simulink model "faultHandling_combined"  (R2018a)
settings: Solver=VariableStepAuto  StartTime=0.0  StopTime=100  FixedStep=1e-2  MaxStep=1e-1  MinStep=1e-6  RelTol=1e-9
undefined symbols (not defined in the file): b, I, I_wheel, K, k_e, k_t, kd, ki, kp, L, magnitude, R
libraries: aausat3_lib x30, dspindex x3, sharedutil x1, library x1
(part 1 of 2)
settings Model: Creator=media  LastModifiedBy=Daniel
settings SolverCC: ZeroCrossAlgorithm=Adaptive  AlgebraicLoopSolver=LineSearch
settings DebuggingCC: MaxConsecutiveZCsMsg=none

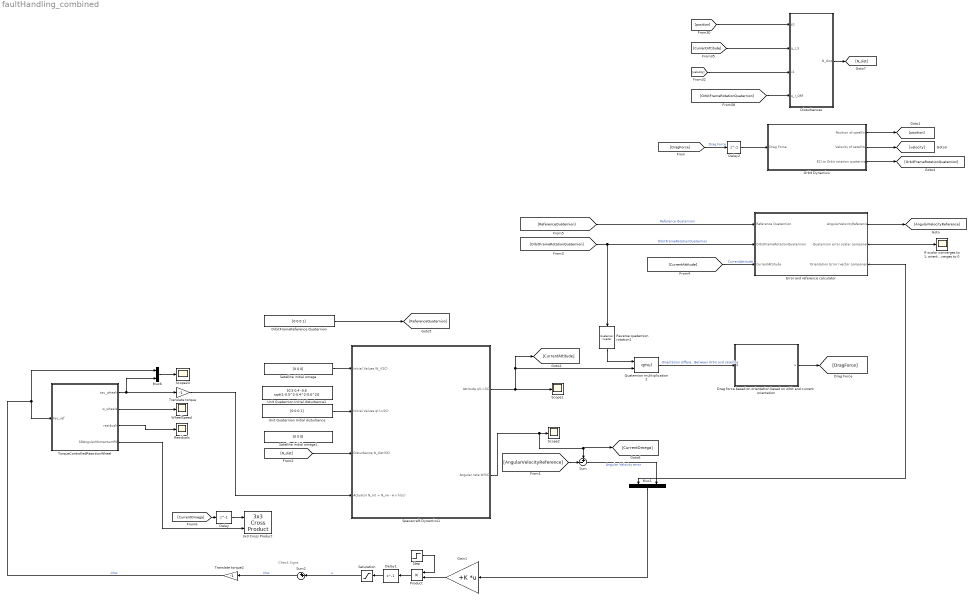
== system faultHandling_combined ==
  note: Check Signs
  3x3 Cross Product : sharedutil/3x3 Cross Product  aMode=aMode
      settings: SourceProductBaseCode=AE
  Delay : Delay  DelayLength=1  InitialCondition=[0;0;0]
  Delay1 : Delay  DelayLength=1  InitialCondition=[0;0;0]
  Delay2 : Delay  DelayLength=1  InitialCondition=0
  Disturbances : Subsystem
  Drag force based on orientation based on orbit and current orientation : Subsystem  TreatAsAtomicUnit=on
  Error and reference calculator : Subsystem
  Gain1 : Gain  Gain=+K  Multiplication=Matrix(K*u)
  "If scalar converges to 1, orientation error converges to 0" : Scope
  Mux1 : Mux  Inputs=2
  Mux6 : Mux  Inputs=2
  Orbit Dynamics : Subsystem
  OrbitFrameReference Quaternion : Constant  Value=[0 0 0 1]
  Product : Product
  Quaternion mulitiplication2 : S-Function  FunctionName=qmul  SFunctionDeploymentMode=off  EnableBusSupport=off
  Residuals : Scope
  Reverse quaternion rotation1 : aausat3_lib/Math Utilities/Quaternion operations/Vector rotation by q/Quaternion inverter
      settings: SourceProductName=AAUSAT3
  Satellite initial omega : Constant  Value=[0 0 0]
  Satellite initial omega1 : Constant  Value=[0 0 0]
  Saturation : Saturate  UpperLimit=2*10^-3  LowerLimit=-2*10^-3
  Scope1 : Scope
  Scope2 : Scope
  Scope24 : Scope
  Spacecraft Dynamics1 : Subsystem  AncestorBlock=spacecraft_dynamics2_lib/Spacecraft Dynamics
  Step : Step  Time=1000  Before=1  After=0  SampleTime=0
  Sum : Sum  Inputs=+-|
  Sum2 : Sum  Inputs=++|
  TorqueControlledReactionWheel : Subsystem
  Translate torque : Gain  Gain=-1
  Translate torque2 : Gain  Gain=-1
  Unit Quaternion Initial disturbance : Constant  Value=[0 0 0 1]
  Unit Quaternion Initial disturbance1 : Constant  Value=[0.5 0.4 -0.6 sqrt(1-0.5^2-0.4^2-0.6^2)]
  WheelSpeed : Scope
  wires:
  Satellite initial omega/1 -> Spacecraft Dynamics1/1(Initial Values W_i(SC))
  Unit Quaternion Initial disturbance/1 -> Spacecraft Dynamics1/2(Initial Values q(I->SC))
  Drag force based on orientation based on orbit and current orientation/1(u) -> [DragForce]
  Spacecraft Dynamics1/2(Angular rate W(SC)) -> [CurrentOmega], Sum/1, Scope2/1
  Quaternion mulitiplication2/1 -> Drag force based on orientation based on orbit and current orientation/1(q)  "Orientation difference Between Orbit and satellite"
  Spacecraft Dynamics1/1(Attitude q(I->SC)) -> [CurrentAttitude], Quaternion mulitiplication2/2, Scope1/1
  Reverse quaternion rotation1/1 -> Quaternion mulitiplication2/1
  [AngularVelocityReference] -> Sum/2
  Sum/1 -> Mux1/2  "Angular Velocity error"
  [velocity] -> Disturbances/3("v1 ")
  Disturbances/1(N_dist) -> [N_dist]
  [OrbitFrameRotationQuaternion] -> Disturbances/4(q_I_ORF)
  [position] -> Disturbances/1("p1 ")
  [CurrentAttitude] -> Disturbances/2("q_I_S ")
  [OrbitFrameRotationQuaternion] -> Reverse quaternion rotation1/1, Error and reference calculator/2(OrbitFrameRotationQuaternion)  "OrbitFrameRotationQuaternion"
  [DragForce] -> Delay2/1  "Drag Force"
  Orbit Dynamics/1(Position of satellite) -> [position]
  Orbit Dynamics/2(Velocity of satellite) -> [velocity]
  Orbit Dynamics/3(ECI to Orbit rotation quaternion) -> [OrbitFrameRotationQuaternion]
  [ReferenceQuaternion] -> Error and reference calculator/1(Reference Quaternion)  "Reference Quaternion"
  [CurrentAttitude] -> Error and reference calculator/3(CurrentAttitude)  "CurrentAttitude"
  Error and reference calculator/1(AngularVelocityReference) -> [AngularVelocityReference]
  Error and reference calculator/2(Quaternion error scalar component) -> "If scalar converges to 1, orientation error converges to 0"/1
  Error and reference calculator/3(Orientation Error (vector component)) -> Mux1/1
  TorqueControlledReactionWheel/2(w_wheels) -> WheelSpeed/1
  TorqueControlledReactionWheel/3(residuals) -> Residuals/1
  Mux6/1 -> Scope24/1
  OrbitFrameReference Quaternion/1 -> [ReferenceQuaternion]
  TorqueControlledReactionWheel/4(3DAngularMomentumRW) -> 3x3 Cross Product/2
  [CurrentOmega] -> Delay/1
  TorqueControlledReactionWheel/1(tau_wheels) -> Mux6/2, Translate torque/1
  Delay/1 -> 3x3 Cross Product/1
  Saturation/1 -> Sum2/2  "u"
  Translate torque2/1 -> Mux6/1, TorqueControlledReactionWheel/1("tau_ref ")  "-Nrw"
  Sum2/1 -> Translate torque2/1  "Nrw"
  Mux1/1 -> Gain1/1
  Gain1/1 -> Product/2
  Product/1 -> Delay1/1
  Step/1 -> Product/1
  [N_dist] -> Spacecraft Dynamics1/3(Disturbance N_dist(SC))
  Translate torque/1 -> Spacecraft Dynamics1/4(Actuator N_mt + N_rw - w x h(sc))
  Delay1/1 -> Saturation/1
  Delay2/1 -> Orbit Dynamics/1(Drag Force)

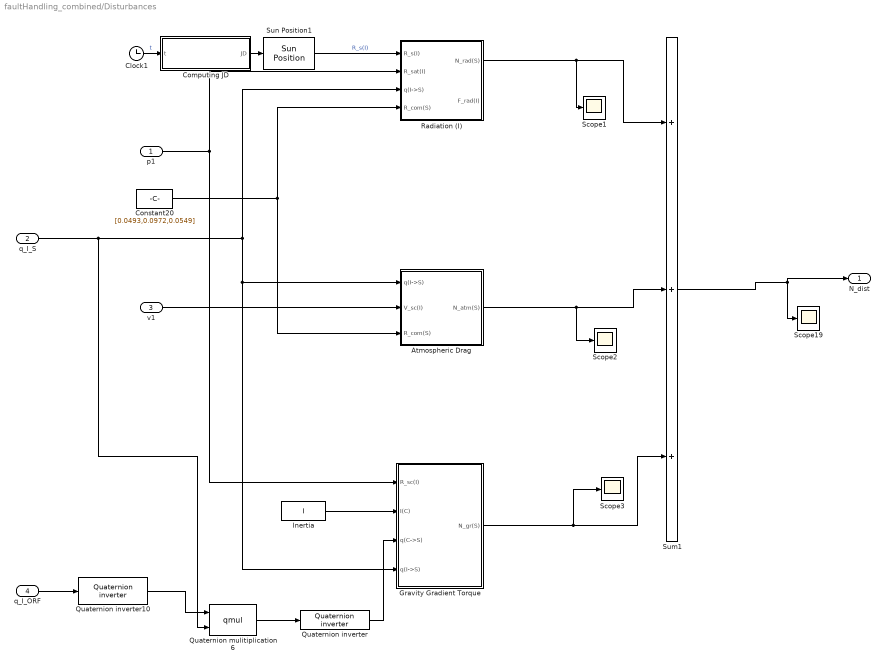
== system faultHandling_combined/Disturbances ==
  "p1 " : Inport
  "q_I_S " : Inport  Port=2
  "v1 " : Inport  Port=3
  q_I_ORF : Inport  Port=4
  Atmospheric Drag : Subsystem  AncestorBlock=aausat3_lib/Disturbances/Atmospheric  mask{Dim=[0.1,0.2,0.1], Cd=2, rho=5e-14}
      mask prompts: Dim "Satellite Dimension [x,y,z][m]:"; Cd "Drag Coefficient [-]:"; rho "Atmospheric Density [kg/m^3]:"
      mask help: Force and torque from the atmospheric drag acting on the satellite.
  Clock1 : Clock
      settings: Decimation=100
  Computing JD : MATLAB Function  TreatAsAtomicUnit=on
  Constant20 : Constant  Value=[0.0493,0.0972,0.0549]
  Gravity Gradient Torque : Subsystem  AncestorBlock=aausat3_lib/Disturbances/Gravity Gradient Torque  mask{G=6.672e-11, M_earth=5.9742e24}
      mask prompts: G "Gravitational Constant [m^3/kgs^2]:"; M_earth "Mass of the Earth [kg]:"
      mask help: Gravitational force applied by the Earth.
  Inertia : Constant  Value=I
  Quaternion inverter : aausat3_lib/Math Utilities/Quaternion operations/Quaternion inverter
      settings: SourceProductName=AAUSAT3
  Quaternion inverter10 : aausat3_lib/Math Utilities/Quaternion operations/Quaternion inverter
      settings: SourceProductName=AAUSAT3
  Quaternion mulitiplication6 : S-Function  FunctionName=qmul  SFunctionDeploymentMode=off  EnableBusSupport=off
  Radiation (I) : Subsystem  AncestorBlock=aausat3_lib/Disturbances/Radiation (I)  mask{Dim=[0.1,0.2,0.1], solar_m_flux=4.5565e-6, solar_absorb_coeff=1.5}
      mask prompts: Dim "Satellite Dimension [x,y,z][m]:"; solar_m_flux "Solar Momentum Flux [kg/ms^2]:"; solar_absorb_coeff "Absorbtion Coefficient [-]:"
      mask help: Solar force and torque acting on the satellite.
  Scope{1..3,19} (4 alike) : Scope
  Sum1 : Sum  Inputs=+++  SaturateOnIntegerOverflow=on
  Sun Position1 : aausat3_lib/Orbit and Ephemeris/Ephemeris/Sun Position
      settings: SourceProductName=AAUSAT3
  N_dist : Outport
  wires:
  Computing JD/1(JD) -> Sun Position1/1
  Sun Position1/1 -> Radiation (I)/1(R_s(I))  "R_s(I)"
  Clock1/1 -> Computing JD/1(t)  "t"
  Sum1/1 -> N_dist/1, Scope19/1
  "q_I_S "/1 -> Quaternion mulitiplication6/2, Radiation (I)/3(q(I->S)), Atmospheric Drag/1(q(I->S)), Gravity Gradient Torque/4(q(I->S))
  Atmospheric Drag/1(N_atm(S)) -> Scope2/1, Sum1/2
  Quaternion inverter10/1 -> Quaternion mulitiplication6/1
  q_I_ORF/1 -> Quaternion inverter10/1
  Quaternion mulitiplication6/1 -> Quaternion inverter/1
  Quaternion inverter/1 -> Gravity Gradient Torque/3(q(C->S))
  "v1 "/1 -> Atmospheric Drag/2(V_sc(I))
  Constant20/1 -> Radiation (I)/4(R_com(S)), Atmospheric Drag/3(R_com(S))
  Inertia/1 -> Gravity Gradient Torque/2(I(C))
  Radiation (I)/1(N_rad(S)) -> Scope1/1, Sum1/1
  Gravity Gradient Torque/1(N_gr(S)) -> Scope3/1, Sum1/3
  "p1 "/1 -> Gravity Gradient Torque/1(R_sc(I)), Radiation (I)/2(R_sat(I))

== system faultHandling_combined/Drag force based on orientation based on orbit and current orientation ==
  q : Inport
  Constant : Constant  Value=[1 0 0]
  Exposed area : aausat3_lib/Other Model Utilities/Exposed area  dim_sat_area=[0.1,0.1,0.1]
      settings: SourceProductName=AAUSAT3
  MATLAB Function : MATLAB Function  TreatAsAtomicUnit=on
  u : Outport
  wires:
  q/1 -> Exposed area/1
  Constant/1 -> Exposed area/2
  Exposed area/1 -> MATLAB Function/1(A)
  MATLAB Function/1(u) -> u/1

== system faultHandling_combined/Error and reference calculator ==
  Reference Quaternion : Inport
  OrbitFrameRotationQuaternion : Inport  Port=2
  CurrentAttitude : Inport  Port=3
  Avoiding Jumps In Quaternion : MATLAB Function  TreatAsAtomicUnit=on
  Demux2 : Demux
  Demux3 : Demux
  Derivative : Derivative
  Gain : Gain  Gain=2
  Mux : Mux  Inputs=3
  Mux2 : Mux  Inputs=3
  Quaternion mulitiplication{,1,3..5} (5 alike) : S-Function  FunctionName=qmul  SFunctionDeploymentMode=off  EnableBusSupport=off
  Reverse quaternion rotation : aausat3_lib/Math Utilities/Quaternion operations/Vector rotation by q/Quaternion inverter
      settings: SourceProductName=AAUSAT3
  Reverse quaternion rotation2 : aausat3_lib/Math Utilities/Quaternion operations/Vector rotation by q/Quaternion inverter
      settings: SourceProductName=AAUSAT3
  Reverse quaternion rotation4 : aausat3_lib/Math Utilities/Quaternion operations/Vector rotation by q/Quaternion inverter
      settings: SourceProductName=AAUSAT3
  AngularVelocityReference : Outport
  Quaternion error scalar component : Outport  Port=2
  Orientation Error (vector component) : Outport  Port=3
  wires:
  CurrentAttitude/1 -> Quaternion mulitiplication1/2
  OrbitFrameRotationQuaternion/1 -> Derivative/1, Reverse quaternion rotation2/1, Quaternion mulitiplication/1
  Quaternion mulitiplication1/1 -> Avoiding Jumps In Quaternion/1(q)  "Orientation Error Quaternion"
  Demux2/4 -> Quaternion error scalar component/1  "Quaternion error scalar component"
  Avoiding Jumps In Quaternion/1(q_continuous) -> Demux2/1
  Quaternion mulitiplication/1 -> Reverse quaternion rotation/1
  Reverse quaternion rotation/1 -> Quaternion mulitiplication1/1
  Demux2/2 -> Mux/2
  Demux2/3 -> Mux/3
  Derivative/1 -> Quaternion mulitiplication3/1
  Quaternion mulitiplication4/1 -> Quaternion mulitiplication5/1
  Reference Quaternion/1 -> Quaternion mulitiplication/2, Quaternion mulitiplication5/2, Reverse quaternion rotation4/1
  Gain/1 -> Quaternion mulitiplication4/2  "Pure Orbit Frame Quaternion"
  Quaternion mulitiplication3/1 -> Gain/1
  Demux3/1 -> Mux2/1
  Demux3/3 -> Mux2/3
  Demux3/2 -> Mux2/2
  Quaternion mulitiplication5/1 -> Demux3/1
  Reverse quaternion rotation4/1 -> Quaternion mulitiplication4/1
  Mux2/1 -> AngularVelocityReference/1  "AngularVelocityReference"
  Reverse quaternion rotation2/1 -> Quaternion mulitiplication3/2
  Demux2/1 -> Mux/1
  Mux/1 -> Orientation Error (vector component)/1  "Orientation Error (vector component)"

== system faultHandling_combined/Orbit Dynamics ==
  Drag Force : Inport
  Constant1 : Constant  Value=[0 0 0]
  Delay : Delay  DelayLength=1  InitialCondition=0
  Inertial frame to Orbit frame Rotation matrix : MATLAB Function  TreatAsAtomicUnit=on
  Initial velocity : Constant  Value=[0 7.5459e+03 0]
  Orbit frame distance : Constant  Value=[7*10^6 0 0]
  Satelllite 1 : S-Function  FunctionName=satDynamics_J2  Parameters=1, 5.9722*10^(24), 6.674*10^(-11), 6371009, 1.08262668*10^-3  SFunctionDeploymentMode=off  EnableBusSupport=off
  matrix_to_quaternion : MATLAB Function  TreatAsAtomicUnit=on
  Position of satellite : Outport
  Velocity of satellite : Outport  Port=2
  ECI to Orbit rotation quaternion : Outport  Port=3
  wires:
  Satelllite 1/2 -> Velocity of satellite/1, Inertial frame to Orbit frame Rotation matrix/2(v)  "Velocity of satellite"
  Drag Force/1 -> Satelllite 1/1
  Constant1/1 -> Satelllite 1/2  "Other Disturbances FORCES - but we only care about torques"
  Orbit frame distance/1 -> Satelllite 1/3  "Radius of orbit in meter"
  Initial velocity/1 -> Satelllite 1/4  "Initial velocity in orbit frame"
  Satelllite 1/1 -> Position of satellite/1, Inertial frame to Orbit frame Rotation matrix/1(p)  "Position of satellite"
  Inertial frame to Orbit frame Rotation matrix/1(rotation_matrix) -> matrix_to_quaternion/1(matrix)
  Delay/1 -> matrix_to_quaternion/2(q_prec)
  matrix_to_quaternion/1(q_I_ORF) -> ECI to Orbit rotation quaternion/1, Delay/1  "ECI to Orbit rotation quaternion"

== system faultHandling_combined/Spacecraft Dynamics1 ==
  Initial Values W_i(SC) : Inport
  Initial Values q(I->SC) : Inport  Port=2
  Disturbance N_dist(SC) : Inport  Port=3
  Actuator N_mt + N_rw - w x h(sc) : Inport  Port=4
  Dummy Nrw input : Constant  Value=[0 0 0]
  "Principal and Body frame is aligned, Principal frame  q(SC->P)" : Constant  Value=[0 0 0 1]
  Reaction wheel initial ang moment : Constant  Value=[0 0 0 ]
  Reverse quaternion rotation : aausat3_lib/Math Utilities/Quaternion operations/Vector rotation by q/Quaternion inverter
      settings: SourceProductName=AAUSAT3
  Rotation of q1 by q1 : aausat3_lib/Math Utilities/Quaternion operations/Rotation of q1 by q2
      settings: SourceProductName=AAUSAT3
  Rotation of q1 by q2 : aausat3_lib/Math Utilities/Quaternion operations/Rotation of q1 by q2
      settings: SourceProductName=AAUSAT3
  S-Function : S-Function  FunctionName=scdynamics3  SFunctionDeploymentMode=off  EnableBusSupport=off
  S-Function1 : S-Function  Commented=on  FunctionName=scdynamics2  SFunctionDeploymentMode=off  EnableBusSupport=off
  Spacecraft Inertia I(P) : Constant  Value=I
  Vector rotation by q{,2..4} (4 alike) : aausat3_lib/Math Utilities/Quaternion operations/Vector rotation by q
      settings: SourceProductName=AAUSAT3
  Attitude q(I->SC) : Outport
  Angular rate W(SC) : Outport  Port=2
  wires:
  S-Function/1 -> Vector rotation by q4/2
  S-Function/3 -> Rotation of q1 by q1/1
  Reaction wheel initial ang moment/1 -> S-Function/2
  Actuator N_mt + N_rw - w x h(sc)/1 -> Vector rotation by q2/2
  Vector rotation by q/1 -> S-Function/1
  Vector rotation by q2/1 -> S-Function/4
  Vector rotation by q3/1 -> S-Function/6
  Disturbance N_dist(SC)/1 -> Vector rotation by q3/2
  Dummy Nrw input/1 -> S-Function/5
  Rotation of q1 by q1/1 -> Attitude q(I->SC)/1
  Spacecraft Inertia I(P)/1 -> S-Function/7
  Rotation of q1 by q2/1 -> S-Function/3
  Vector rotation by q4/1 -> Angular rate W(SC)/1
  Initial Values q(I->SC)/1 -> Rotation of q1 by q2/1
  "Principal and Body frame is aligned, Principal frame  q(SC->P)"/1 -> Rotation of q1 by q2/2, Vector rotation by q/1, Vector rotation by q2/1, Vector rotation by q3/1, Reverse quaternion rotation/1
  Initial Values W_i(SC)/1 -> Vector rotation by q/2
  Reverse quaternion rotation/1 -> Vector rotation by q4/1, Rotation of q1 by q1/2

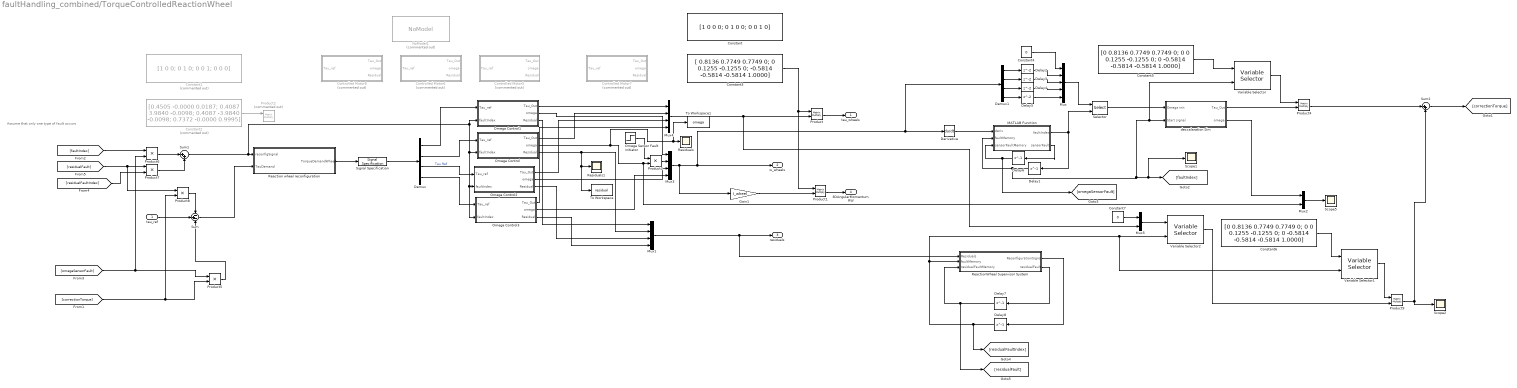
== system faultHandling_combined/TorqueControlledReactionWheel ==
  note: Assume that only one type of fault occurs
  "tau_ref " : Inport
  Constant : Constant  Value=[1 0 0 0; 0 1 0 0; 0 0 1 0]
  Constant1 : Constant  Commented=on  Value=[1 0 0; 0 1 0; 0 0 1; 0 0 0]
  Constant2 : Constant  Commented=on  Value=|
      | [0.4505   -0.0000    0.0187;
      |     0.4087    3.9840   -0.0098;
      |     0.4087   -3.9840   -0.0098;
      |     0.7372   -0.0000    0.9995]
  Constant3 : Constant  Value=|
      | [    0.8136    0.7749    0.7749         0;
      |          0    0.1255   -0.1255         0;
      |    -0.5814   -0.5814   -0.5814    1.0000]
  Constant4 : Constant  Value=0
  Constant5 : Constant  Value=|
      | [0    0.8136    0.7749    0.7749         0;
      |  0        0    0.1255   -0.1255         0;
      |  0  -0.5814   -0.5814   -0.5814    1.0000]
  Constant6 : Constant  Value=|
      | [0    0.8136    0.7749    0.7749         0;
      |  0        0    0.1255   -0.1255         0;
      |  0  -0.5814   -0.5814   -0.5814    1.0000]
  Constant7 : Constant  Value=0
  Controlled Motor5 : Subsystem  Commented=on
  Controlled Motor6 : Subsystem  Commented=on
  Controlled Motor7 : Subsystem  Commented=on
  Controlled Motor8 : Subsystem  Commented=on
  Delay{1,6..8} (4 alike) : Delay  DelayLength=1  InitialCondition=0
  Delay{2..5} (4 alike) : Delay  InitialCondition=0
  Demux : Demux
  Demux1 : Demux
  Derivative : Derivative
  Gain1 : Gain  Gain=I_wheel
  MATLAB Function : MATLAB Function  TreatAsAtomicUnit=on
  Mux : Mux  Inputs=5
  Mux1 : Mux
  Mux2 : Mux  Inputs=2
  Mux3 : Mux
  Mux4 : Mux
  Mux5 : Mux  Inputs=2
  NoModel1 : library/Reaction Wheel Models/NoModel  Commented=on
  Omega Control : Subsystem
  Omega Control1 : Subsystem
  Omega Control2 : Subsystem
  Omega Control3 : Subsystem
  Omega Sensor Fault initiator : Step  Time=1000  Before=1  After=0  SampleTime=0
  Product{,1,4,9} (4 alike) : Product  Multiplication=Matrix(*)
  Product2 : Product  Commented=on  Multiplication=Matrix(*)
  Product{3,5..8} (5 alike) : Product
  Reaction wheel reconfiguration : MATLAB Function  TreatAsAtomicUnit=on
  ReactionWheel Supervisor System : MATLAB Function  TreatAsAtomicUnit=on
  Residuals : Scope
  Residuals1 : Scope
  Scope1 : Scope
  Scope2 : Scope
  Scope5 : Scope
  Selector : Selector  IndexMode=Zero-based  InputPortWidth=5  IndexOptions=Index vector (port)  Indices=[1 3]  OutputSizes=1
  Signal Specification : SignalSpecification  Dimensions=4
  Sum : Sum  Inputs=-+-
  Sum1 : Sum  Inputs=|++
  Sum2 : Sum  Inputs=|++
  To Workspace : ToWorkspace  VariableName=residual  SaveFormat=Timeseries  SampleTime=-1
  To Workspace1 : ToWorkspace  VariableName=omega  SaveFormat=Timeseries  SampleTime=-1
  Variable Selector : dspindex/Variable Selector  NumInputs=1  rowsOrCols=Columns  IdxMode=Variable  Elements=[1 3]  ZerOneIdxMode=Zero-based  errmode=Clip Index  FillMode=on  FillValues=0
  Variable Selector1 : dspindex/Variable Selector  NumInputs=1  rowsOrCols=Columns  IdxMode=Variable  Elements=[1 3]  ZerOneIdxMode=Zero-based  errmode=Clip Index  FillMode=on  FillValues=0
  Variable Selector2 : dspindex/Variable Selector  NumInputs=1  rowsOrCols=Rows  IdxMode=Variable  Elements=[1 3]  ZerOneIdxMode=Zero-based  errmode=Clip Index  FillMode=on  FillValues=0
  deccalaration Sim : Subsystem
  tau_wheels : Outport
  w_wheels : Outport  Port=2
  residuals : Outport  Port=3
  3DAngularMomentumRW : Outport  Port=4
  wires:
  Demux/4 -> Omega Control3/1(Tau_ref)
  Omega Control3/1("Tau_Out ") -> Mux4/4
  Omega Control3/2(omega) -> Mux3/4
  Demux/3 -> Omega Control2/1(Tau_ref)  "Tau Ref"
  Demux/2 -> Omega Control/1(Tau_ref)
  Omega Control/1("Tau_Out ") -> Mux4/2
  Omega Control2/1("Tau_Out ") -> Mux4/3
  Omega Control1/2(omega) -> Mux3/1
  Omega Control2/2(omega) -> Mux3/3
  Omega Control1/3(Residual) -> Mux1/1
  Omega Control/3(Residual) -> To Workspace/1, Residuals1/1, Mux1/2
  Omega Control2/3(Residual) -> Mux1/3
  Omega Control3/3(Residual) -> Mux1/4
  Mux1/1 -> ReactionWheel Supervisor System/1(Residuals), residuals/1
  Omega Control1/1("Tau_Out ") -> Mux4/1
  Gain1/1 -> Product1/2
  Product/1 -> tau_wheels/1
  Product1/1 -> 3DAngularMomentumRW/1
  Demux/1 -> Omega Control1/1(Tau_ref)
  Constant3/1 -> Product1/1, Product/1
  Product3/1 -> Mux3/2
  Omega Control/2(omega) -> To Workspace1/1, Residuals/1, Mux2/2, Product3/2
  Derivative/1 -> MATLAB Function/1(deriv)
  Mux3/1 -> Gain1/1, Derivative/1, Demux1/1, w_wheels/1
  Selector/1 -> deccalaration Sim/1(Omega init)
  deccalaration Sim/2(omega) -> Mux2/1
  Demux1/1 -> Delay2/1
  Demux1/4 -> Delay5/1
  Demux1/3 -> Delay4/1
  Demux1/2 -> Delay3/1
  Delay5/1 -> Mux/5
  Delay4/1 -> Mux/4
  Delay3/1 -> Mux/3
  Delay2/1 -> Mux/2
  Constant4/1 -> Mux/1
  Mux/1 -> Selector/1
  Constant5/1 -> Variable Selector/1
  deccalaration Sim/1("Tau_Out ") -> Product4/2
  Constant2/1 -> Product2/1
  Sum1/1 -> Omega Control1/2(faultIndex), Omega Control2/2(faultIndex), Omega Control3/2(faultIndex), Omega Control/2(faultIndex), Reaction wheel reconfiguration/1(reconfigSignal)
  Variable Selector/1 -> Product4/1
  Signal Specification/1 -> Demux/1
  Reaction wheel reconfiguration/1(TorqueDemandWheel) -> Signal Specification/1
  Sum/1 -> Reaction wheel reconfiguration/2(TauDemand)
  Mux2/1 -> Scope5/1
  Omega Sensor Fault initiator/1 -> Product3/1
  MATLAB Function/2(sensorFault) -> Delay6/1
  Delay6/1 -> [omegaSensorFault], MATLAB Function/3(sensorFaultMemory)
  Delay1/1 -> MATLAB Function/2(faultMemory), Variable Selector/2, deccalaration Sim/2(Start signal), Scope1/1, [faultIndex]
  [correctionTorque] -> Product8/2, Product5/2
  [omegaSensorFault] -> Product5/1, Product6/2
  ReactionWheel Supervisor System/1(ReconfigurationSignal) -> Delay8/1
  MATLAB Function/1(faultIndex) -> Delay1/1, Selector/2
  Delay7/1 -> [residualFault], ReactionWheel Supervisor System/3(residualFaultMemory)
  ReactionWheel Supervisor System/2(residualFault) -> Delay7/1
  Delay8/1 -> [residualFaultIndex], ReactionWheel Supervisor System/2(faultMemory), Variable Selector1/2, Variable Selector2/2
  [faultIndex] -> Product6/1
  Product6/1 -> Sum1/1
  [residualFaultIndex] -> Product7/2
  [residualFault] -> Product8/1, Product7/1
  Product7/1 -> Sum1/2
  "tau_ref "/1 -> Sum/2
  Product5/1 -> Sum/3
  Product8/1 -> Sum/1
  Sum2/1 -> [correctionTorque]
  Product4/1 -> Sum2/1
  Constant6/1 -> Variable Selector1/1
  Variable Selector1/1 -> Product9/1
  Variable Selector2/1 -> Product9/2
  Mux4/1 -> Mux5/2, Product/2
  Product9/1 -> Sum2/2, Scope2/1
  Mux5/1 -> Variable Selector2/1
  Constant7/1 -> Mux5/1

== system faultHandling_combined/Disturbances/Atmospheric Drag ==
  q(I->S) : Inport
  V_sc(I) : Inport  Port=2
  R_com(S) : Inport  Port=3
  C_D : Constant  Value=Cd
  Cross Product : aausat3_lib/Math Utilities/Vector operations/Cross Product
      settings: SourceProductName=AAUSAT3
  Density : Constant  Value=rho
  Dimensions : Constant  Value=Dim
  Exposed area : aausat3_lib/Other Model Utilities/Exposed area  dim_sat_area=[0.1,0.2,0.1]
      settings: SourceProductName=AAUSAT3
  Gain : Gain  Gain=-1/2  SaturateOnIntegerOverflow=on  OutDataTypeStr=Inherit: Same as input  ParamDataTypeStr=Inherit: Same as input
  Gain1 : Gain  Gain=1/2  SaturateOnIntegerOverflow=on  OutDataTypeStr=Inherit: Same as input  ParamDataTypeStr=Inherit: Same as input
  Product{1..4} (4 alike) : Product  SaturateOnIntegerOverflow=on  OutDataTypeStr=Inherit: Same as first input
  Sum : Sum  Inputs=|-+
  To unit vector : aausat3_lib/Math Utilities/Vector operations/To unit vector
      settings: SourceProductName=AAUSAT3
  Vector rotation by q : aausat3_lib/Math Utilities/Quaternion operations/Vector rotation by q
      settings: SourceProductName=AAUSAT3
  math operation : Math  Operator=magnitude^2  SaturateOnIntegerOverflow=on
  N_atm(S) : Outport
  wires:
  Sum/1 -> Cross Product/1
  R_com(S)/1 -> Sum/1  "Center of Mass"
  Gain1/1 -> Sum/2  "Geometric Center"
  Dimensions/1 -> Gain1/1
  Vector rotation by q/1 -> Cross Product/2
  Gain/1 -> Vector rotation by q/2
  Product4/1 -> Gain/1
  q(I->S)/1 -> Exposed area/1, Vector rotation by q/1
  Density/1 -> Product3/2
  Product2/1 -> Product3/1
  Product1/1 -> Product2/2
  math operation/1 -> Product1/1
  To unit vector/1 -> Product1/2
  V_sc(I)/1 -> Exposed area/2, To unit vector/1, math operation/1
  Exposed area/1 -> Product2/1
  C_D/1 -> Product4/1
  Product3/1 -> Product4/2
  Cross Product/1 -> N_atm(S)/1

== system faultHandling_combined/Disturbances/Gravity Gradient Torque ==
  note: To principal frame
  R_sc(I) : Inport
  I(C) : Inport  Port=2
  q(C->S) : Inport  Port=3
  q(I->S) : Inport  Port=4
  " " : Subsystem
  3*GM : Gain  Gain=3*G*M_earth  SaturateOnIntegerOverflow=on  OutDataTypeStr=Inherit: Same as input  ParamDataTypeStr=Inherit: Same as input
  Constant : Constant  Value=3
  Constant1 : Constant  Value=[1 0 0;0 1 0;0 0 1]
  Constant2 : Constant  Value=[1 1 1]  VectorParams1D=off
  Cross Product : aausat3_lib/Math Utilities/Vector operations/Cross Product
      settings: SourceProductName=AAUSAT3
  Dot roduct : DotProduct  InputSameDT=on  OutDataTypeStr=Inherit: Inherit via internal rule
  Product : Product  Multiplication=Matrix(*)  SaturateOnIntegerOverflow=on  OutDataTypeStr=Inherit: Same as first input
  Product1 : Product  SaturateOnIntegerOverflow=on  OutDataTypeStr=Inherit: Same as first input
  Product2 : Product  Multiplication=Matrix(*)  SaturateOnIntegerOverflow=on  OutDataTypeStr=Inherit: Same as first input
  Product3 : Product  SaturateOnIntegerOverflow=on  OutDataTypeStr=Inherit: Same as first input
  R : Math  Operator=pow  SaturateOnIntegerOverflow=on
  To unit vector : aausat3_lib/Math Utilities/Vector operations/To unit vector
      settings: SourceProductName=AAUSAT3
  Vector rotation by q : aausat3_lib/Math Utilities/Quaternion operations/Vector rotation by q
      settings: SourceProductName=AAUSAT3
  inv : Math  Operator=reciprocal  SaturateOnIntegerOverflow=on
  inv1 : Math  Operator=sqrt  SaturateOnIntegerOverflow=on
  N_gr(S) : Outport
  wires:
  Cross Product/1 -> Vector rotation by q/2
  Dot roduct/1 -> inv1/1
  Product3/1 -> N_gr(S)/1
  R/1 -> 3*GM/1
  inv/1 -> R/1
  inv1/1 -> inv/1
  Constant/1 -> R/2
  To unit vector/1 -> Product/2, Cross Product/1
  q(C->S)/1 -> " "/1(q(C->SC)), Vector rotation by q/1
  q(I->S)/1 -> " "/2("q(I -> SC)")
  " "/1(R_sc(C)) -> To unit vector/1
  Product1/1 -> Product/1
  Product/1 -> Cross Product/2
  I(C)/1 -> Product2/1
  Constant2/1 -> Product2/2
  Product2/1 -> Product1/1
  Constant1/1 -> Product1/2
  R_sc(I)/1 -> Dot roduct/2, Dot roduct/1, " "/3(R_sc(I))
  3*GM/1 -> Product3/1
  Vector rotation by q/1 -> Product3/2

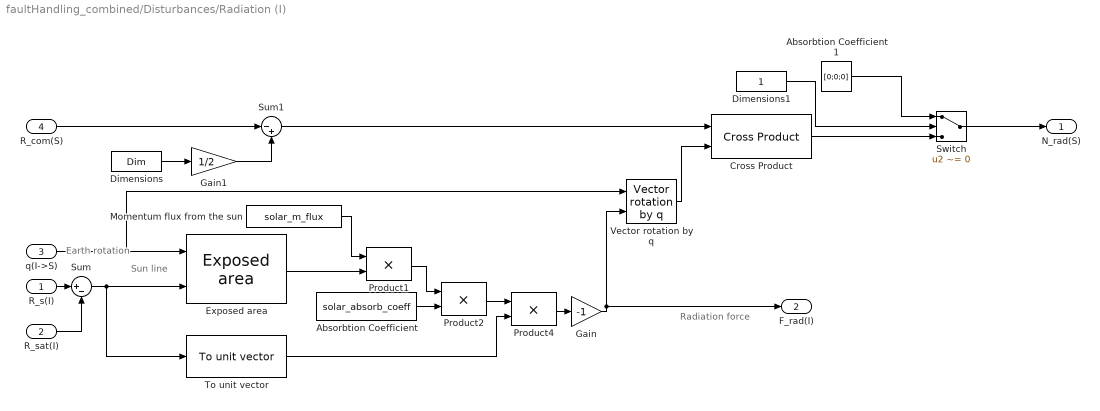
== system faultHandling_combined/Disturbances/Radiation (I) ==
  note: Sun line
  note: Earth rotation
  note: Radiation force
  R_s(I) : Inport
  R_sat(I) : Inport  Port=2
  q(I->S) : Inport  Port=3
  R_com(S) : Inport  Port=4
  Absorbtion Coefficient : Constant  Value=solar_absorb_coeff
  Absorbtion Coefficient1 : Constant  Value=[0;0;0]
  Cross Product : aausat3_lib/Math Utilities/Vector operations/Cross Product
      settings: SourceProductName=AAUSAT3
  Dimensions : Constant  Value=Dim
  Dimensions1 : Constant
  Exposed area : aausat3_lib/Other Model Utilities/Exposed area  dim_sat_area=[0.1,0.2,0.1]
      settings: SourceProductName=AAUSAT3
  Gain : Gain  Gain=-1  SaturateOnIntegerOverflow=on  OutDataTypeStr=Inherit: Same as input  ParamDataTypeStr=Inherit: Same as input
  Gain1 : Gain  Gain=1/2  SaturateOnIntegerOverflow=on  OutDataTypeStr=Inherit: Same as input  ParamDataTypeStr=Inherit: Same as input
  Momentum flux from the sun : Constant  Value=solar_m_flux
  Product1 : Product  SaturateOnIntegerOverflow=on  OutDataTypeStr=Inherit: Same as first input
  Product2 : Product  SaturateOnIntegerOverflow=on  OutDataTypeStr=Inherit: Same as first input
  Product4 : Product  SaturateOnIntegerOverflow=on  OutDataTypeStr=Inherit: Same as first input
  Sum : Sum  Inputs=|+-  SaturateOnIntegerOverflow=on
  Sum1 : Sum  Inputs=|-+
  Switch : Switch  Criteria=u2 ~= 0
  To unit vector : aausat3_lib/Math Utilities/Vector operations/To unit vector
      settings: SourceProductName=AAUSAT3
  Vector rotation by q : aausat3_lib/Math Utilities/Quaternion operations/Vector rotation by q
      settings: SourceProductName=AAUSAT3
  N_rad(S) : Outport
  F_rad(I) : Outport  Port=2
  wires:
  Absorbtion Coefficient1/1 -> Switch/1
  Switch/1 -> N_rad(S)/1
  R_s(I)/1 -> Sum/1
  R_sat(I)/1 -> Sum/2
  q(I->S)/1 -> Exposed area/1, Vector rotation by q/1
  Sum/1 -> Exposed area/2, To unit vector/1
  Product1/1 -> Product2/1
  Absorbtion Coefficient/1 -> Product2/2
  Product2/1 -> Product4/1
  To unit vector/1 -> Product4/2
  Product4/1 -> Gain/1
  Gain/1 -> Vector rotation by q/2, F_rad(I)/1
  Vector rotation by q/1 -> Cross Product/2
  Exposed area/1 -> Product1/2
  Momentum flux from the sun/1 -> Product1/1
  Cross Product/1 -> Switch/3
  Dimensions/1 -> Gain1/1
  R_com(S)/1 -> Sum1/1
  Gain1/1 -> Sum1/2
  Sum1/1 -> Cross Product/1
  Dimensions1/1 -> Switch/2

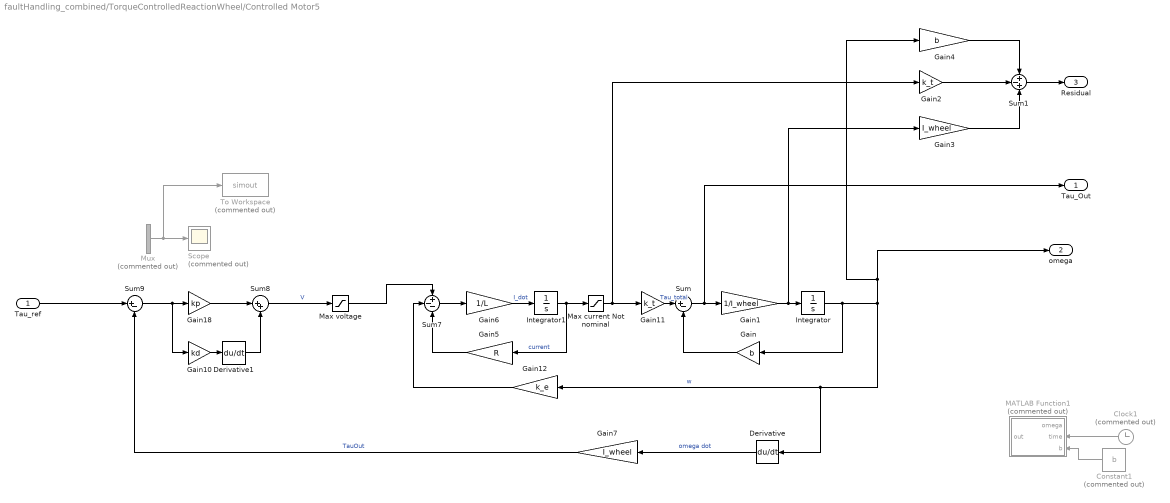
== system faultHandling_combined/TorqueControlledReactionWheel/Controlled Motor5 ==
  Tau_ref : Inport
  Clock1 : Clock  Commented=on
  Constant1 : Constant  Commented=on  Value=b
  Derivative : Derivative
  Derivative1 : Derivative
  Gain : Gain  Gain=b
  Gain1 : Gain  Gain=1/I_wheel
  Gain10 : Gain  Gain=kd
  Gain11 : Gain  Gain=k_t
  Gain12 : Gain  Gain=k_e
  Gain18 : Gain  Gain=kp
  Gain2 : Gain  Gain=k_t
  Gain3 : Gain  Gain=I_wheel
  Gain4 : Gain  Gain=b
  Gain5 : Gain  Gain=R
  Gain6 : Gain  Gain=1/L
  Gain7 : Gain  Gain=I_wheel
  Integrator : Integrator
  Integrator1 : Integrator
  MATLAB Function1 : MATLAB Function  Commented=on  TreatAsAtomicUnit=on
  Max current Not nominal : Saturate  UpperLimit=1.5  LowerLimit=-1.5
  Max voltage : Saturate  UpperLimit=6  LowerLimit=-6
  Mux : Mux  Commented=on  Inputs=2
  Scope : Scope  Commented=on
  Sum : Sum  Inputs=|+-
  Sum1 : Sum  Inputs=+-+
  Sum7 : Sum  Inputs=+--
  Sum8 : Sum  Inputs=|++
  Sum9 : Sum  Inputs=|+-
  To Workspace : ToWorkspace  Commented=on  VariableName=simout  SaveFormat=Timeseries  SampleTime=-1
  "Tau_Out " : Outport
  omega : Outport  Port=2
  Residual : Outport  Port=3
  wires:
  Max current Not nominal/1 -> Gain2/1, Gain11/1
  Derivative/1 -> Gain7/1  "omega dot"
  Gain18/1 -> Sum8/1
  Gain6/1 -> Integrator1/1  "I_dot"
  Sum7/1 -> Gain6/1
  Integrator/1 -> Gain/1, Gain4/1, omega/1, Derivative/1, Gain12/1  "w"
  Sum9/1 -> Gain10/1, Gain18/1
  Gain10/1 -> Derivative1/1
  Gain11/1 -> Sum/1  "Tau_total"
  Gain2/1 -> Sum1/2
  Gain4/1 -> Sum1/1
  Gain3/1 -> Sum1/3
  Sum1/1 -> Residual/1
  Sum8/1 -> Max voltage/1  "V"
  Tau_ref/1 -> Sum9/1
  Sum/1 -> "Tau_Out "/1, Gain1/1
  Gain1/1 -> Gain3/1, Integrator/1
  Max voltage/1 -> Sum7/1
  Gain12/1 -> Sum7/2
  Gain5/1 -> Sum7/3
  Integrator1/1 -> Gain5/1, Max current Not nominal/1  "current"
  Mux/1 -> To Workspace/1, Scope/1
  Constant1/1 -> MATLAB Function1/3(b)
  Clock1/1 -> MATLAB Function1/2(time)
  Gain/1 -> Sum/2
  Gain7/1 -> Sum9/2  "TauOut"
  Derivative1/1 -> Sum8/2

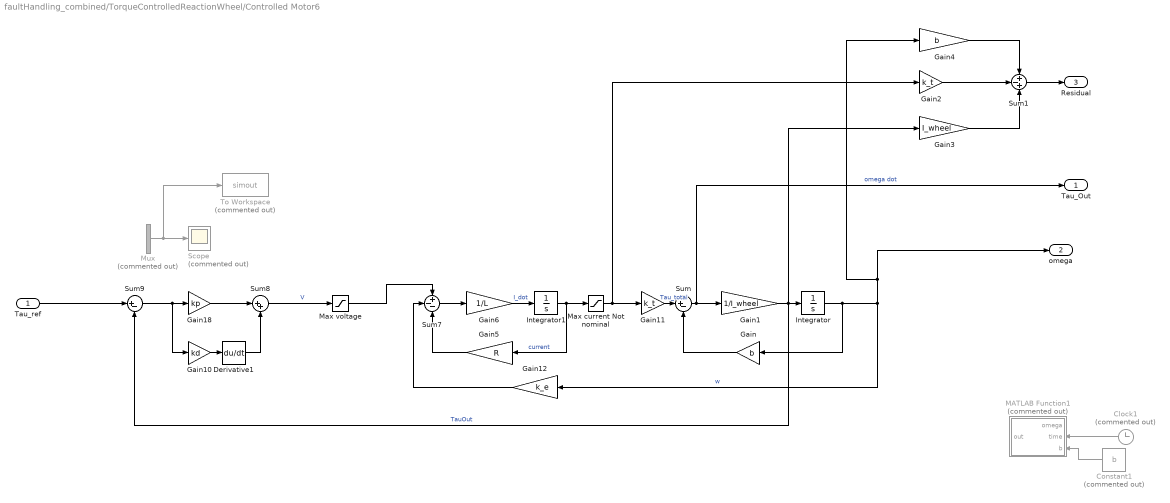
== system faultHandling_combined/TorqueControlledReactionWheel/Controlled Motor6 ==
  Tau_ref : Inport
  Clock1 : Clock  Commented=on
  Constant1 : Constant  Commented=on  Value=b
  Derivative1 : Derivative
  Gain : Gain  Gain=b
  Gain1 : Gain  Gain=1/I_wheel
  Gain10 : Gain  Gain=kd
  Gain11 : Gain  Gain=k_t
  Gain12 : Gain  Gain=k_e
  Gain18 : Gain  Gain=kp
  Gain2 : Gain  Gain=k_t
  Gain3 : Gain  Gain=I_wheel
  Gain4 : Gain  Gain=b
  Gain5 : Gain  Gain=R
  Gain6 : Gain  Gain=1/L
  Integrator : Integrator
  Integrator1 : Integrator
  MATLAB Function1 : MATLAB Function  Commented=on  TreatAsAtomicUnit=on
  Max current Not nominal : Saturate  UpperLimit=1.5  LowerLimit=-1.5
  Max voltage : Saturate  UpperLimit=6  LowerLimit=-6
  Mux : Mux  Commented=on  Inputs=2
  Scope : Scope  Commented=on
  Sum : Sum  Inputs=|+-
  Sum1 : Sum  Inputs=+-+
  Sum7 : Sum  Inputs=+--
  Sum8 : Sum  Inputs=|++
  Sum9 : Sum  Inputs=|+-
  To Workspace : ToWorkspace  Commented=on  VariableName=simout  SaveFormat=Timeseries  SampleTime=-1
  "Tau_Out " : Outport
  omega : Outport  Port=2
  Residual : Outport  Port=3
  wires:
  Max current Not nominal/1 -> Gain2/1, Gain11/1
  Sum/1 -> Gain1/1, "Tau_Out "/1  "omega dot"
  Gain18/1 -> Sum8/1
  Gain6/1 -> Integrator1/1  "I_dot"
  Sum7/1 -> Gain6/1
  Integrator/1 -> Gain/1, Gain4/1, omega/1, Gain12/1  "w"
  Sum9/1 -> Gain10/1, Gain18/1
  Gain10/1 -> Derivative1/1
  Gain11/1 -> Sum/1  "Tau_total"
  Gain2/1 -> Sum1/2
  Gain4/1 -> Sum1/1
  Gain3/1 -> Sum1/3
  Sum1/1 -> Residual/1
  Sum8/1 -> Max voltage/1  "V"
  Tau_ref/1 -> Sum9/1
  Max voltage/1 -> Sum7/1
  Gain12/1 -> Sum7/2
  Gain5/1 -> Sum7/3
  Integrator1/1 -> Gain5/1, Max current Not nominal/1  "current"
  Mux/1 -> To Workspace/1, Scope/1
  Constant1/1 -> MATLAB Function1/3(b)
  Clock1/1 -> MATLAB Function1/2(time)
  Gain/1 -> Sum/2
  Gain1/1 -> Sum9/2, Gain3/1, Integrator/1  "TauOut"
  Derivative1/1 -> Sum8/2

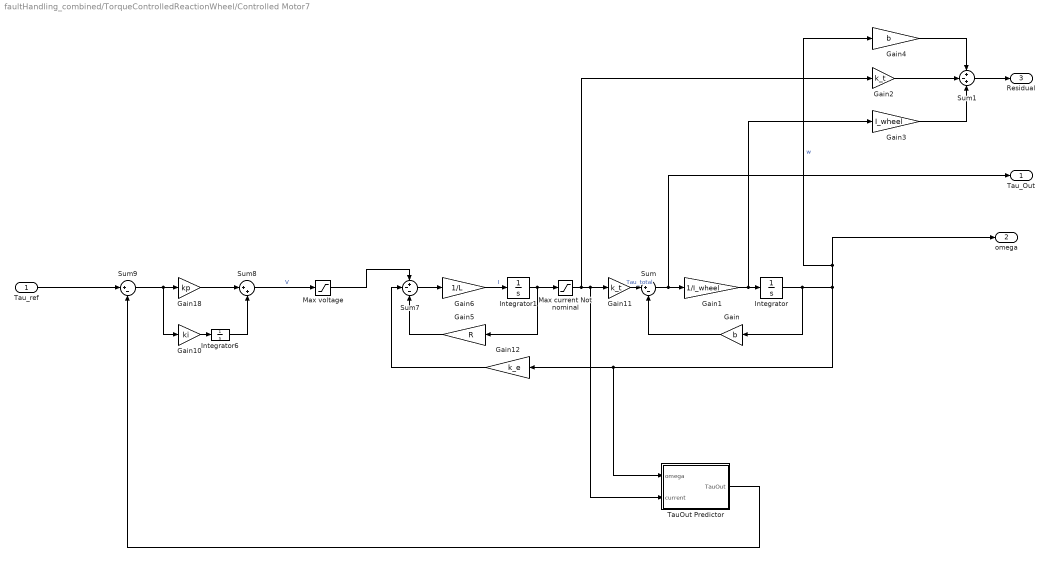
== system faultHandling_combined/TorqueControlledReactionWheel/Controlled Motor7 ==
  Tau_ref : Inport
  Gain : Gain  Gain=b
  Gain1 : Gain  Gain=1/I_wheel
  Gain10 : Gain  Gain=ki
  Gain11 : Gain  Gain=k_t
  Gain12 : Gain  Gain=k_e
  Gain18 : Gain  Gain=kp
  Gain2 : Gain  Gain=k_t
  Gain3 : Gain  Gain=I_wheel
  Gain4 : Gain  Gain=b
  Gain5 : Gain  Gain=R
  Gain6 : Gain  Gain=1/L
  Integrator : Integrator
  Integrator1 : Integrator
  Integrator6 : Integrator
  Max current Not nominal : Saturate  UpperLimit=1.5  LowerLimit=-1.5
  Max voltage : Saturate  UpperLimit=6  LowerLimit=-6
  Sum : Sum  Inputs=|+-
  Sum1 : Sum  Inputs=+-+
  Sum7 : Sum  Inputs=+--
  Sum8 : Sum  Inputs=|++
  Sum9 : Sum  Inputs=|+-
  TauOut Predictor : Subsystem
  "Tau_Out " : Outport
  omega : Outport  Port=2
  Residual : Outport  Port=3
  wires:
  Max current Not nominal/1 -> Gain2/1, Gain11/1, TauOut Predictor/2(current)
  TauOut Predictor/1(TauOut) -> Sum9/2
  Gain18/1 -> Sum8/1
  Integrator6/1 -> Sum8/2
  Gain6/1 -> Integrator1/1  "I"
  Sum7/1 -> Gain6/1
  Integrator/1 -> Gain/1, Gain4/1, omega/1, TauOut Predictor/1(omega), Gain12/1  "w"
  Sum9/1 -> Gain10/1, Gain18/1
  Gain10/1 -> Integrator6/1
  Gain11/1 -> Sum/1  "Tau_total"
  Gain2/1 -> Sum1/2
  Gain4/1 -> Sum1/1
  Gain3/1 -> Sum1/3
  Sum1/1 -> Residual/1
  Sum8/1 -> Max voltage/1  "V"
  Tau_ref/1 -> Sum9/1
  Gain/1 -> Sum/2
  Sum/1 -> "Tau_Out "/1, Gain1/1
  Gain1/1 -> Gain3/1, Integrator/1
  Max voltage/1 -> Sum7/1
  Gain12/1 -> Sum7/2
  Gain5/1 -> Sum7/3
  Integrator1/1 -> Gain5/1, Max current Not nominal/1

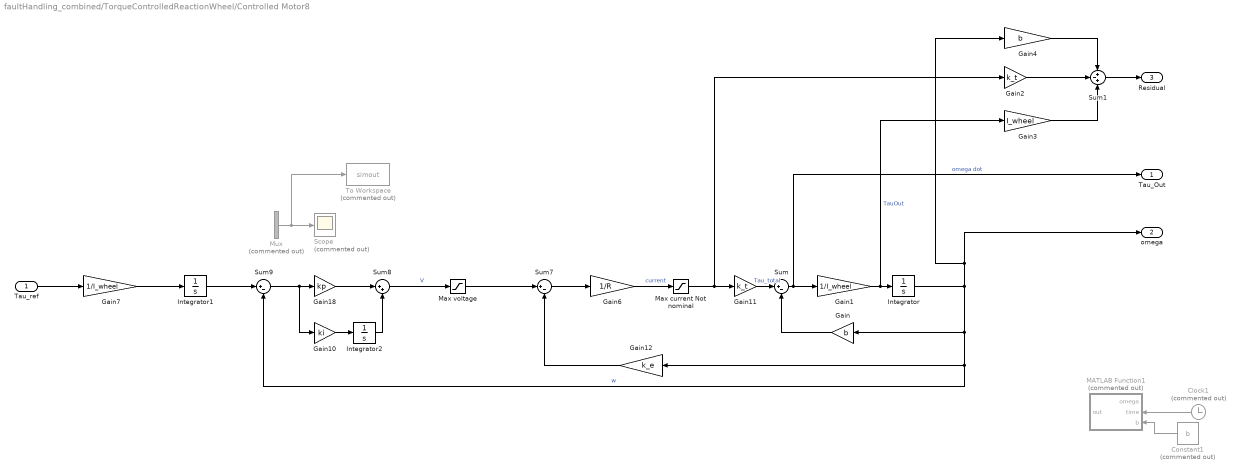
== system faultHandling_combined/TorqueControlledReactionWheel/Controlled Motor8 ==
  Tau_ref : Inport
  Clock1 : Clock  Commented=on
  Constant1 : Constant  Commented=on  Value=b
  Gain : Gain  Gain=b
  Gain1 : Gain  Gain=1/I_wheel
  Gain10 : Gain  Gain=ki
  Gain11 : Gain  Gain=k_t
  Gain12 : Gain  Gain=k_e
  Gain18 : Gain  Gain=kp
  Gain2 : Gain  Gain=k_t
  Gain3 : Gain  Gain=I_wheel
  Gain4 : Gain  Gain=b
  Gain6 : Gain  Gain=1/R
  Gain7 : Gain  Gain=1/I_wheel
  Integrator : Integrator
  Integrator1 : Integrator
  Integrator2 : Integrator
  MATLAB Function1 : MATLAB Function  Commented=on  TreatAsAtomicUnit=on
  Max current Not nominal : Saturate  UpperLimit=1.5  LowerLimit=-1.5
  Max voltage : Saturate  UpperLimit=6  LowerLimit=-6
  Mux : Mux  Commented=on  Inputs=2
  Scope : Scope  Commented=on
  Sum : Sum  Inputs=|+-
  Sum1 : Sum  Inputs=+-+
  Sum7 : Sum  Inputs=|+-
  Sum8 : Sum  Inputs=|++
  Sum9 : Sum  Inputs=|+-
  To Workspace : ToWorkspace  Commented=on  VariableName=simout  SaveFormat=Timeseries  SampleTime=-1
  "Tau_Out " : Outport
  omega : Outport  Port=2
  Residual : Outport  Port=3
  wires:
  Max current Not nominal/1 -> Gain2/1, Gain11/1
  Sum/1 -> Gain1/1, "Tau_Out "/1  "omega dot"
  Gain18/1 -> Sum8/1
  Integrator/1 -> Gain/1, Gain12/1, Sum9/2, Gain4/1, omega/1  "w"
  Sum9/1 -> Gain10/1, Gain18/1
  Gain10/1 -> Integrator2/1
  Gain11/1 -> Sum/1  "Tau_total"
  Gain2/1 -> Sum1/2
  Gain4/1 -> Sum1/1
  Gain3/1 -> Sum1/3
  Sum1/1 -> Residual/1
  Sum8/1 -> Max voltage/1  "V"
  Max voltage/1 -> Sum7/1
  Gain12/1 -> Sum7/2
  Gain6/1 -> Max current Not nominal/1  "current"
  Mux/1 -> To Workspace/1, Scope/1
  Constant1/1 -> MATLAB Function1/3(b)
  Clock1/1 -> MATLAB Function1/2(time)
  Gain/1 -> Sum/2
  Gain1/1 -> Gain3/1, Integrator/1  "TauOut"
  Integrator2/1 -> Sum8/2
  Tau_ref/1 -> Gain7/1
  Sum7/1 -> Gain6/1
  Gain7/1 -> Integrator1/1
  Integrator1/1 -> Sum9/1

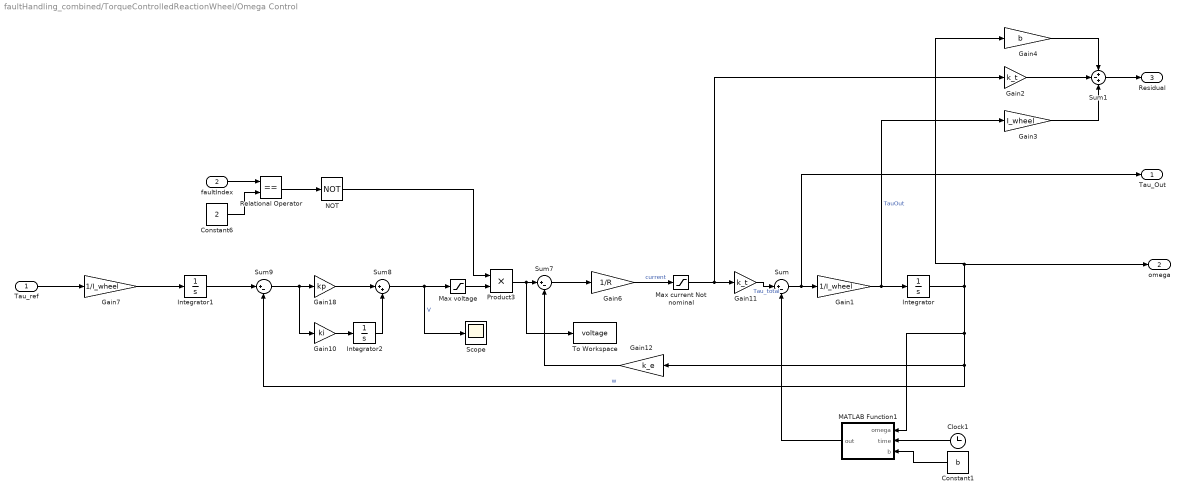
== system faultHandling_combined/TorqueControlledReactionWheel/Omega Control ==
  Tau_ref : Inport
  faultIndex : Inport  Port=2
  Clock1 : Clock
  Constant1 : Constant  Value=b
  Constant6 : Constant  Value=2
  Gain1 : Gain  Gain=1/I_wheel
  Gain10 : Gain  Gain=ki
  Gain11 : Gain  Gain=k_t
  Gain12 : Gain  Gain=k_e
  Gain18 : Gain  Gain=kp
  Gain2 : Gain  Gain=k_t
  Gain3 : Gain  Gain=I_wheel
  Gain4 : Gain  Gain=b
  Gain6 : Gain  Gain=1/R
  Gain7 : Gain  Gain=1/I_wheel
  Integrator : Integrator
  Integrator1 : Integrator
  Integrator2 : Integrator
  MATLAB Function1 : MATLAB Function  TreatAsAtomicUnit=on
  Max current Not nominal : Saturate  UpperLimit=1.5  LowerLimit=-1.5
  Max voltage : Saturate  UpperLimit=6  LowerLimit=-6
  NOT : Logic  Operator=NOT  IconShape=distinctive  AllPortsSameDT=off  OutDataTypeStr=boolean
  Product3 : Product
  Relational Operator : RelationalOperator  Operator===  OutDataTypeStr=boolean  ZeroCross=off  RndMeth=Simplest
  Scope : Scope
  Sum : Sum  Inputs=|+-
  Sum1 : Sum  Inputs=+-+
  Sum7 : Sum  Inputs=|+-
  Sum8 : Sum  Inputs=|++
  Sum9 : Sum  Inputs=|+-
  To Workspace : ToWorkspace  VariableName=voltage  SaveFormat=Timeseries  SampleTime=-1
  "Tau_Out " : Outport
  omega : Outport  Port=2
  Residual : Outport  Port=3
  wires:
  Max current Not nominal/1 -> Gain11/1, Gain2/1
  Sum/1 -> Gain1/1, "Tau_Out "/1
  Gain18/1 -> Sum8/1
  Integrator/1 -> MATLAB Function1/1(omega), Gain12/1, Sum9/2, Gain4/1, omega/1  "w"
  Sum9/1 -> Gain10/1, Gain18/1
  Gain10/1 -> Integrator2/1
  Gain11/1 -> Sum/1  "Tau_total"
  Gain2/1 -> Sum1/2
  Gain4/1 -> Sum1/1
  Gain3/1 -> Sum1/3
  Sum1/1 -> Residual/1
  Sum8/1 -> Scope/1, Max voltage/1  "V"
  Gain12/1 -> Sum7/2
  Gain6/1 -> Max current Not nominal/1  "current"
  Constant1/1 -> MATLAB Function1/3(b)
  Clock1/1 -> MATLAB Function1/2(time)
  MATLAB Function1/1(out) -> Sum/2
  Gain1/1 -> Gain3/1, Integrator/1  "TauOut"
  Integrator2/1 -> Sum8/2
  Tau_ref/1 -> Gain7/1
  Sum7/1 -> Gain6/1
  Gain7/1 -> Integrator1/1
  Integrator1/1 -> Sum9/1
  Product3/1 -> To Workspace/1, Sum7/1
  Max voltage/1 -> Product3/2
  NOT/1 -> Product3/1
  Relational Operator/1 -> NOT/1
  Constant6/1 -> Relational Operator/2
  faultIndex/1 -> Relational Operator/1

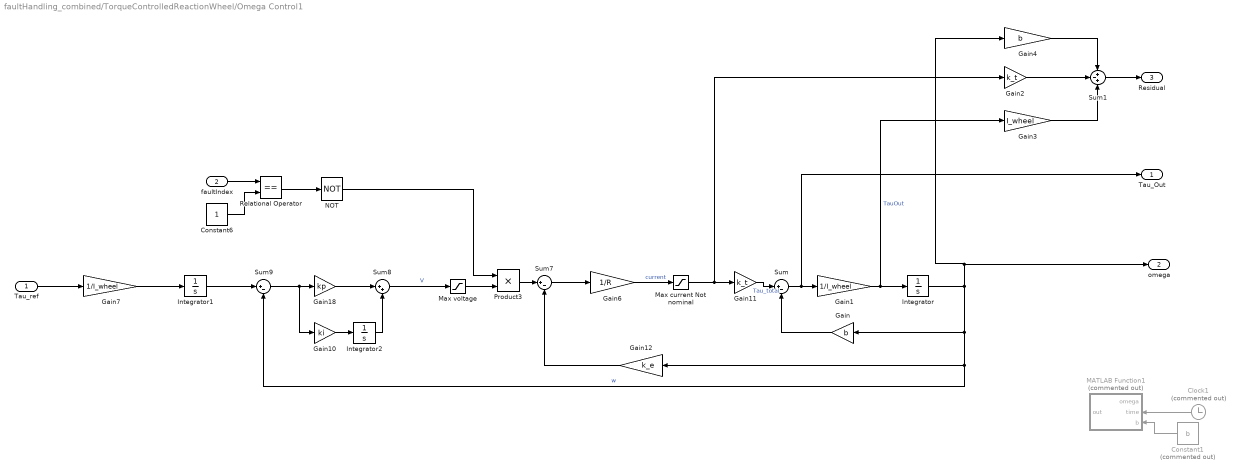
== system faultHandling_combined/TorqueControlledReactionWheel/Omega Control1 ==
  Tau_ref : Inport
  faultIndex : Inport  Port=2
  Clock1 : Clock  Commented=on
  Constant1 : Constant  Commented=on  Value=b
  Constant6 : Constant
  Gain : Gain  Gain=b
  Gain1 : Gain  Gain=1/I_wheel
  Gain10 : Gain  Gain=ki
  Gain11 : Gain  Gain=k_t
  Gain12 : Gain  Gain=k_e
  Gain18 : Gain  Gain=kp
  Gain2 : Gain  Gain=k_t
  Gain3 : Gain  Gain=I_wheel
  Gain4 : Gain  Gain=b
  Gain6 : Gain  Gain=1/R
  Gain7 : Gain  Gain=1/I_wheel
  Integrator : Integrator
  Integrator1 : Integrator
  Integrator2 : Integrator
  MATLAB Function1 : MATLAB Function  Commented=on  TreatAsAtomicUnit=on
  Max current Not nominal : Saturate  UpperLimit=1.5  LowerLimit=-1.5
  Max voltage : Saturate  UpperLimit=6  LowerLimit=-6
  NOT : Logic  Operator=NOT  IconShape=distinctive  AllPortsSameDT=off  OutDataTypeStr=boolean
  Product3 : Product
  Relational Operator : RelationalOperator  Operator===  OutDataTypeStr=boolean  ZeroCross=off  RndMeth=Simplest
  Sum : Sum  Inputs=|+-
  Sum1 : Sum  Inputs=+-+
  Sum7 : Sum  Inputs=|+-
  Sum8 : Sum  Inputs=|++
  Sum9 : Sum  Inputs=|+-
  "Tau_Out " : Outport
  omega : Outport  Port=2
  Residual : Outport  Port=3
  wires:
  Max current Not nominal/1 -> Gain11/1, Gain2/1
  Sum/1 -> Gain1/1, "Tau_Out "/1
  Gain18/1 -> Sum8/1
  Integrator/1 -> Gain/1, Gain12/1, Sum9/2, Gain4/1, omega/1  "w"
  Sum9/1 -> Gain10/1, Gain18/1
  Gain10/1 -> Integrator2/1
  Gain11/1 -> Sum/1  "Tau_total"
  Gain2/1 -> Sum1/2
  Gain4/1 -> Sum1/1
  Gain3/1 -> Sum1/3
  Sum1/1 -> Residual/1
  Sum8/1 -> Max voltage/1  "V"
  Gain12/1 -> Sum7/2
  Gain6/1 -> Max current Not nominal/1  "current"
  Constant1/1 -> MATLAB Function1/3(b)
  Clock1/1 -> MATLAB Function1/2(time)
  Gain/1 -> Sum/2
  Gain1/1 -> Gain3/1, Integrator/1  "TauOut"
  Integrator2/1 -> Sum8/2
  Tau_ref/1 -> Gain7/1
  Sum7/1 -> Gain6/1
  Gain7/1 -> Integrator1/1
  Integrator1/1 -> Sum9/1
  Product3/1 -> Sum7/1
  Max voltage/1 -> Product3/2
  NOT/1 -> Product3/1
  Relational Operator/1 -> NOT/1
  Constant6/1 -> Relational Operator/2
  faultIndex/1 -> Relational Operator/1

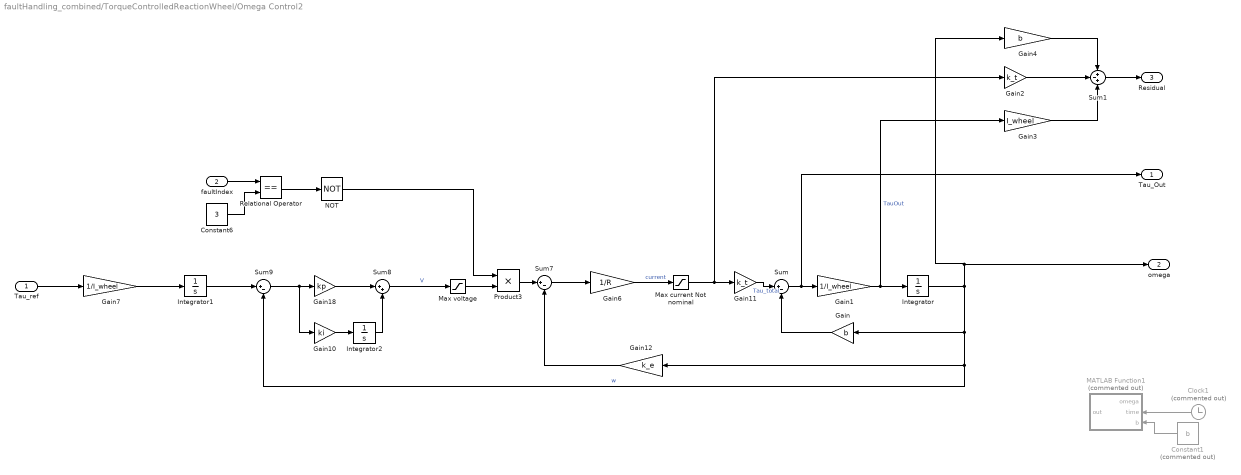
== system faultHandling_combined/TorqueControlledReactionWheel/Omega Control2 ==
  Tau_ref : Inport
  faultIndex : Inport  Port=2
  Clock1 : Clock  Commented=on
  Constant1 : Constant  Commented=on  Value=b
  Constant6 : Constant  Value=3
  Gain : Gain  Gain=b
  Gain1 : Gain  Gain=1/I_wheel
  Gain10 : Gain  Gain=ki
  Gain11 : Gain  Gain=k_t
  Gain12 : Gain  Gain=k_e
  Gain18 : Gain  Gain=kp
  Gain2 : Gain  Gain=k_t
  Gain3 : Gain  Gain=I_wheel
  Gain4 : Gain  Gain=b
  Gain6 : Gain  Gain=1/R
  Gain7 : Gain  Gain=1/I_wheel
  Integrator : Integrator
  Integrator1 : Integrator
  Integrator2 : Integrator
  MATLAB Function1 : MATLAB Function  Commented=on  TreatAsAtomicUnit=on
  Max current Not nominal : Saturate  UpperLimit=1.5  LowerLimit=-1.5
  Max voltage : Saturate  UpperLimit=6  LowerLimit=-6
  NOT : Logic  Operator=NOT  IconShape=distinctive  AllPortsSameDT=off  OutDataTypeStr=boolean
  Product3 : Product
  Relational Operator : RelationalOperator  Operator===  OutDataTypeStr=boolean  ZeroCross=off  RndMeth=Simplest
  Sum : Sum  Inputs=|+-
  Sum1 : Sum  Inputs=+-+
  Sum7 : Sum  Inputs=|+-
  Sum8 : Sum  Inputs=|++
  Sum9 : Sum  Inputs=|+-
  "Tau_Out " : Outport
  omega : Outport  Port=2
  Residual : Outport  Port=3
  wires:
  Max current Not nominal/1 -> Gain11/1, Gain2/1
  Sum/1 -> Gain1/1, "Tau_Out "/1
  Gain18/1 -> Sum8/1
  Integrator/1 -> Gain/1, Gain12/1, Sum9/2, Gain4/1, omega/1  "w"
  Sum9/1 -> Gain10/1, Gain18/1
  Gain10/1 -> Integrator2/1
  Gain11/1 -> Sum/1  "Tau_total"
  Gain2/1 -> Sum1/2
  Gain4/1 -> Sum1/1
  Gain3/1 -> Sum1/3
  Sum1/1 -> Residual/1
  Sum8/1 -> Max voltage/1  "V"
  Gain12/1 -> Sum7/2
  Gain6/1 -> Max current Not nominal/1  "current"
  Constant1/1 -> MATLAB Function1/3(b)
  Clock1/1 -> MATLAB Function1/2(time)
  Gain/1 -> Sum/2
  Gain1/1 -> Gain3/1, Integrator/1  "TauOut"
  Integrator2/1 -> Sum8/2
  Tau_ref/1 -> Gain7/1
  Sum7/1 -> Gain6/1
  Gain7/1 -> Integrator1/1
  Integrator1/1 -> Sum9/1
  Product3/1 -> Sum7/1
  Max voltage/1 -> Product3/2
  NOT/1 -> Product3/1
  Relational Operator/1 -> NOT/1
  Constant6/1 -> Relational Operator/2
  faultIndex/1 -> Relational Operator/1

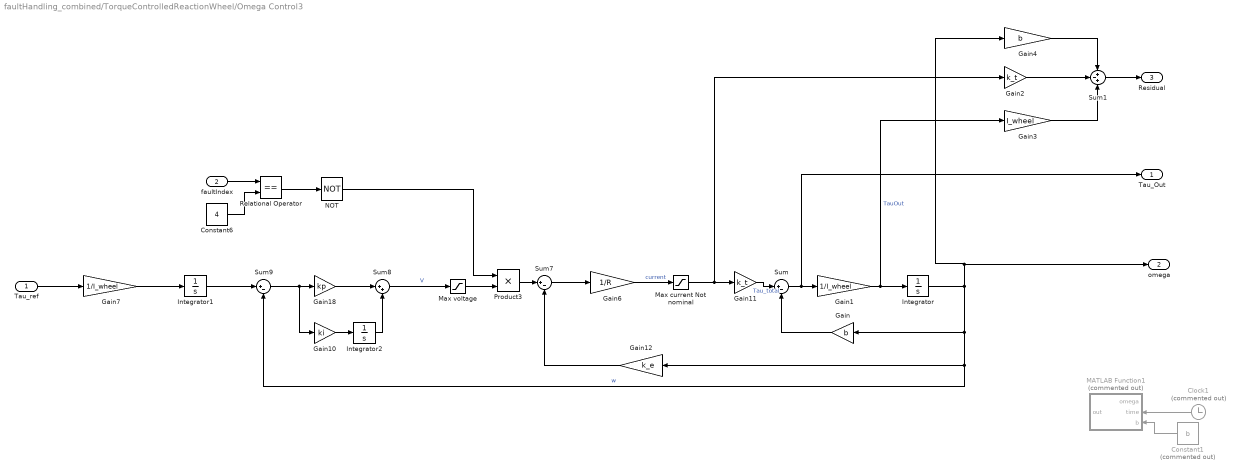
== system faultHandling_combined/TorqueControlledReactionWheel/Omega Control3 ==
  Tau_ref : Inport
  faultIndex : Inport  Port=2
  Clock1 : Clock  Commented=on
  Constant1 : Constant  Commented=on  Value=b
  Constant6 : Constant  Value=4
  Gain : Gain  Gain=b
  Gain1 : Gain  Gain=1/I_wheel
  Gain10 : Gain  Gain=ki
  Gain11 : Gain  Gain=k_t
  Gain12 : Gain  Gain=k_e
  Gain18 : Gain  Gain=kp
  Gain2 : Gain  Gain=k_t
  Gain3 : Gain  Gain=I_wheel
  Gain4 : Gain  Gain=b
  Gain6 : Gain  Gain=1/R
  Gain7 : Gain  Gain=1/I_wheel
  Integrator : Integrator
  Integrator1 : Integrator
  Integrator2 : Integrator
  MATLAB Function1 : MATLAB Function  Commented=on  TreatAsAtomicUnit=on
  Max current Not nominal : Saturate  UpperLimit=1.5  LowerLimit=-1.5
  Max voltage : Saturate  UpperLimit=6  LowerLimit=-6
  NOT : Logic  Operator=NOT  IconShape=distinctive  AllPortsSameDT=off  OutDataTypeStr=boolean
  Product3 : Product
  Relational Operator : RelationalOperator  Operator===  OutDataTypeStr=boolean  ZeroCross=off  RndMeth=Simplest
  Sum : Sum  Inputs=|+-
  Sum1 : Sum  Inputs=+-+
  Sum7 : Sum  Inputs=|+-
  Sum8 : Sum  Inputs=|++
  Sum9 : Sum  Inputs=|+-
  "Tau_Out " : Outport
  omega : Outport  Port=2
  Residual : Outport  Port=3
  wires:
  Max current Not nominal/1 -> Gain11/1, Gain2/1
  Sum/1 -> Gain1/1, "Tau_Out "/1
  Gain18/1 -> Sum8/1
  Integrator/1 -> Gain/1, Gain12/1, Sum9/2, Gain4/1, omega/1  "w"
  Sum9/1 -> Gain10/1, Gain18/1
  Gain10/1 -> Integrator2/1
  Gain11/1 -> Sum/1  "Tau_total"
  Gain2/1 -> Sum1/2
  Gain4/1 -> Sum1/1
  Gain3/1 -> Sum1/3
  Sum1/1 -> Residual/1
  Sum8/1 -> Max voltage/1  "V"
  Gain12/1 -> Sum7/2
  Gain6/1 -> Max current Not nominal/1  "current"
  Constant1/1 -> MATLAB Function1/3(b)
  Clock1/1 -> MATLAB Function1/2(time)
  Gain/1 -> Sum/2
  Gain1/1 -> Gain3/1, Integrator/1  "TauOut"
  Integrator2/1 -> Sum8/2
  Tau_ref/1 -> Gain7/1
  Sum7/1 -> Gain6/1
  Gain7/1 -> Integrator1/1
  Integrator1/1 -> Sum9/1
  Product3/1 -> Sum7/1
  Max voltage/1 -> Product3/2
  NOT/1 -> Product3/1
  Relational Operator/1 -> NOT/1
  Constant6/1 -> Relational Operator/2
  faultIndex/1 -> Relational Operator/1

== system faultHandling_combined/TorqueControlledReactionWheel/deccalaration Sim ==
  Omega init : Inport
  Start signal : Inport  Port=2
  Gain : Gain  Gain=b
  Gain1 : Gain  Gain=1/I_wheel
  Gain11 : Gain  Gain=k_t
  Gain12 : Gain  Gain=k_e
  Gain2 : Gain  Gain=-1
  Gain6 : Gain  Gain=1/R
  Integrator : Integrator  ExternalReset=rising  InitialConditionSource=external
  Max current Not nominal : Saturate  UpperLimit=1.5  LowerLimit=-1.5
  Sum : Sum  Inputs=|+-
  "Tau_Out " : Outport
  omega : Outport  Port=2
  wires:
  Max current Not nominal/1 -> Gain11/1
  Sum/1 -> Gain1/1, "Tau_Out "/1  "omega dot"
  Integrator/1 -> omega/1, Gain/1, Gain12/1  "w"
  Gain11/1 -> Sum/1  "Tau_total"
  Gain6/1 -> Max current Not nominal/1  "current"
  Gain/1 -> Sum/2
  Gain1/1 -> Integrator/1  "TauOut"
  Gain12/1 -> Gain2/1
  Omega init/1 -> Integrator/3
  Start signal/1 -> Integrator/2
  Gain2/1 -> Gain6/1

== system faultHandling_combined/Disturbances/Gravity Gradient Torque/  ==
  q(C->SC) : Inport
  "q(I -> SC)" : Inport  Port=2
  R_sc(I) : Inport  Port=3
  Quaternion inverter : aausat3_lib/Math Utilities/Quaternion operations/Quaternion inverter
      settings: SourceProductName=AAUSAT3
  Rotation of q1 by q2 : aausat3_lib/Math Utilities/Quaternion operations/Rotation of q1 by q2
      settings: SourceProductName=AAUSAT3
  To unit vector : aausat3_lib/Math Utilities/Vector operations/To unit vector
      settings: SourceProductName=AAUSAT3
  Vector rotation by q : aausat3_lib/Math Utilities/Quaternion operations/Vector rotation by q
      settings: SourceProductName=AAUSAT3
  R_sc(C) : Outport
  wires:
  "q(I -> SC)"/1 -> Rotation of q1 by q2/1
  q(C->SC)/1 -> Quaternion inverter/1
  Quaternion inverter/1 -> Rotation of q1 by q2/2
  R_sc(I)/1 -> To unit vector/1
  Rotation of q1 by q2/1 -> Vector rotation by q/1
  To unit vector/1 -> Vector rotation by q/2
  Vector rotation by q/1 -> R_sc(C)/1

== system faultHandling_combined/TorqueControlledReactionWheel/Controlled Motor7/TauOut Predictor ==
  omega : Inport
  current : Inport  Port=2
  Constant : Constant  Value=k_t
  Constant1 : Constant  Value=b
  Output torque estimator : MATLAB Function  TreatAsAtomicUnit=on
  TauOut : Outport
  wires:
  Output torque estimator/1(TauOut) -> TauOut/1
  Constant1/1 -> Output torque estimator/3(b)
  Constant/1 -> Output torque estimator/2(k_t)
  current/1 -> Output torque estimator/1(i)
  omega/1 -> Output torque estimator/4(omega)

== matlab function faultHandling_combined/Orbit Dynamics/matrix_to_quaternion ==
  data: matrix input; q_I_ORF output; q_prec input
function q_I_ORF = fcn(matrix,q_prec)

    tr = matrix(1,1) + matrix(2,2) + matrix(3,3);

    if( tr > 0 ) 
    	S = sqrt(tr+1.0) * 2;
        a = 0.25 * S;
        b = (matrix(3,2) - matrix(2,3)) / S;
        c = (matrix(1,3) - matrix(3,1)) / S; 
        d = (matrix(2,1) - matrix(1,2)) / S; 
    elseif( (matrix(1,1) > matrix(2,2) ) && ( matrix(1,1) > matrix(3,3) ) )
        S = sqrt(1.0 + matrix(1,1) - matrix(2,2) - matrix(3,3)) * 2;
        a = (matrix(3,2) - matrix(2,3)) / S;
        if( a < 0 )
            a = -a;
            S = -S;
        end
        b = 0.25 * S;
        c = (matrix(1,2) + matrix(2,1)) / S; 
        d = (matrix(1,3) + matrix(3,1)) / S; 
    elseif( matrix(2,2) > matrix(3,3) ) 
        S = sqrt(1.0 + matrix(2,2) - matrix(1,1) - matrix(3,3)) * 2;
        a = (matrix(1,3) - matrix(3,1)) / S;
        if( a < 0 )
            a = -a;
            S = -S;
        end
        b = (matrix(1,2) + matrix(2,1)) / S; 
        c = 0.25 * S;
        d = (matrix(2,3) + matrix(3,2)) / S; 
    else
        S = sqrt(1.0 + matrix(3,3) - matrix(1,1) - matrix(2,2)) * 2;
        a = (matrix(2,1) - matrix(1,2)) / S;
        if( a < 0 )
            a = -a;
            S = -S;
        end
        b = (matrix(1,3) + matrix(3,1)) / S;
        c = (matrix(2,3) + matrix(3,2)) / S;
        d = 0.25 * S;
    end
    
    q_I_ORF = [b,c,d,a]';
    
    
    if( (abs(q_I_ORF(1) - q_prec(1)) > 1) || (abs(q_I_ORF(2) - q_prec(2)) > 1) || (abs(q_I_ORF(3) - q_prec(3)) > 1) || (abs(q_I_ORF(4) - q_prec(4)) > 1) )
        q_I_ORF = - q_I_ORF;
    end
end

== matlab function faultHandling_combined/Orbit Dynamics/Inertial frame to Orbit frame Rotation matrix ==
  data: p input; rotation_matrix output; v input
function rotation_matrix = fcn(p,v)

    y_ORF = -p/norm(p);
    z_ORF = cross(v,y_ORF)/norm(cross(v,y_ORF));
    x_ORF = cross(y_ORF,z_ORF);
    
    rotation_matrix = [x_ORF, y_ORF, z_ORF];

== matlab function faultHandling_combined/Error and reference calculator/Avoiding Jumps In Quaternion ==
  data: q input; q_continuous output
function q_continuous = fcn(q)

   q_continuous = q;
   if(q(4) < 0)
       q_continuous = -q;
   end
   
    
end

== matlab function faultHandling_combined/TorqueControlledReactionWheel/MATLAB Function ==
  data: deriv input; faultIndex output; faultMemory input; sensorFaultMemory input; sensorFault output
function [faultIndex, sensorFault]  = fcn(deriv, faultMemory, sensorFaultMemory)

sensorFault = sensorFaultMemory;

if(faultMemory ~= 0)
    faultIndex = faultMemory;
else
    fault_index = abs(deriv) > 1000; % adjustable threshold
    [maxVal, faultIndex] = max(fault_index);
    if(maxVal == 0)
        faultIndex = 0;
    else
        sensorFault = 1;
    end
end

== matlab function faultHandling_combined/TorqueControlledReactionWheel/Omega Control/MATLAB Function1 ==
  data: omega input; out output; time input; b input
function out = fcn(omega, time, b)

out = omega*b;

if(time > 20)
   out = 2*omega*b;
end

== matlab function faultHandling_combined/TorqueControlledReactionWheel/Omega Control1/MATLAB Function1 ==
  data: omega input; out output; time input; b input
function out = fcn(omega, time, b)

out = omega*b;

% if(time > 30)
%    out = 2*omega*b;
% end
